simulink model "LQR_test"  (R2016a)
settings: Solver=VariableStepAuto  SolverMode=SingleTasking  StartTime=0.0  StopTime=1.5  MaxStep=1e-2  RelTol=1e-3
undefined symbols (not defined in the file): A, B, K
settings Model: Creator=edzel  LastModifiedBy=edzel
settings DataIOCC: ReturnWorkspaceOutputs=on
settings DebuggingCC: UnconnectedInputMsg=none  UnconnectedOutputMsg=none  UnconnectedLineMsg=none  SFUnexpectedBacktrackingDiag=error  SFNoUnconditionalDefaultTransitionDiag=error
settings ModelReferenceCC: EnableRefExpFcnMdlSchedulingChecks=off
settings SFSimCC: SimUseLocalCustomCode=on
settings RTWCC: Description=Generic Real-Time Target  RTWUseLocalCustomCode=on
settings GRTTargetCC: TargetLangStandard=C99 (ISO)
settings ConfigComp: CovMetricSettings=dwe  CovSaveCumulativeToWorkspaceVar=off  CovSaveSingleToWorkspaceVar=off  CovExternalEMLEnable=on

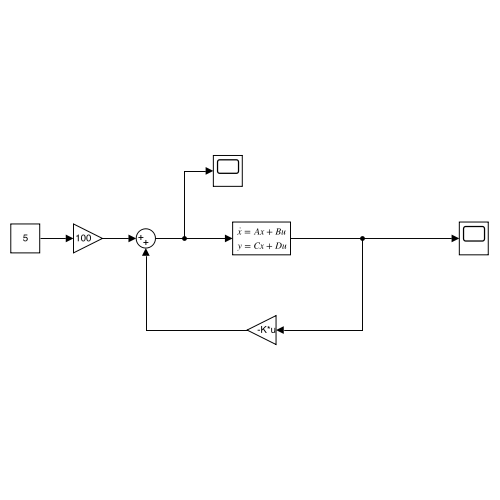
[thumbnail: Simulink's stored preview of the top-level diagram]
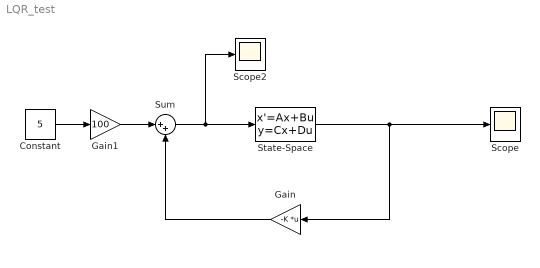
== system LQR_test ==
  Constant : Constant  Value=5
  Gain : Gain  Gain=-K  Multiplication=Matrix(K*u)
  Gain1 : Gain  Gain=100
  Scope : Scope
  Scope2 : Scope
  State-Space : StateSpace  A=A  B=B  C=eye(2)  D=[0; 0]  X0=0
  Sum : Sum  Inputs=|++
  wires:
  State-Space/1 -> Gain/1, Scope/1
  Gain/1 -> Sum/2
  Sum/1 -> Scope2/1, State-Space/1
  Constant/1 -> Gain1/1
  Gain1/1 -> Sum/1
